simulink model "flash_model1"  (R2014b)
settings: Solver=FixedStepDiscrete  SolverMode=SingleTasking  StartTime=0.0  StopTime=10.0  FixedStep=.1  RelTol=1e-3
settings Model: SimulationMode=external  Creator=wildcat  LastModifiedBy=aodell
settings DataIOCC: SaveOutput=off  SignalLogging=off  SaveTime=off
settings SFSimCC: SimCustomHeaderCode=|
  | #include "/Users/aodell/Google Drive/Documents/MATLAB/test_sim/mycfiles/motorboard.h"
  | #include "/Users/aodell/Google Drive/Documents/MATLAB/test_sim/mycfiles/mot.h"
  | #include "/Users/aodell/Google Drive/Documents/MATLAB/test_sim/mycfiles/util.h"
  | #include "/Users/aodell/Google Drive/Documents/MATLAB/test_sim/mycfiles/gpio.h"
  | #include "/Users/aodell/Google Drive/Documents/MATLAB/test_sim/mycfiles/type.h"
settings SFSimCC: SimUserSources=|
  | "/Users/aodell/Google Drive/Documents/MATLAB/test_sim/mycfiles/motorboard.c"
  | "/Users/aodell/Google Drive/Documents/MATLAB/test_sim/mycfiles/mot.c"
  | "/Users/aodell/Google Drive/Documents/MATLAB/test_sim/mycfiles/util.c"
  | "/Users/aodell/Google Drive/Documents/MATLAB/test_sim/mycfiles/gpio.c"
settings RTWCC: GenCodeOnly=on  TargetLang=C++
settings GRTTargetCC: MatFileLogging=off  ExtMode=on  ExtModeMexArgs='192.168.1.1' 1 17725

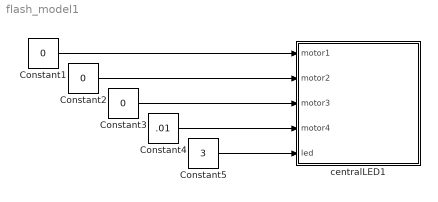
== system flash_model1 ==
  Constant1 : Constant  Value=0
  Constant2 : Constant  Value=0
  Constant3 : Constant  Value=0
  Constant4 : Constant  Value=.01
  Constant5 : Constant  Value=3
  centralLED1 : MATLAB Function  TreatAsAtomicUnit=on
  wires:
  Constant1/1 -> centralLED1/1(motor1)
  Constant2/1 -> centralLED1/2(motor2)
  Constant3/1 -> centralLED1/3(motor3)
  Constant4/1 -> centralLED1/4(motor4)
  Constant5/1 -> centralLED1/5(led)

== matlab function flash_model1/centralLED1 ==
  data: motor1 input; motor2 input; motor3 input; motor4 input; led input
function motorController(motor1,motor2,motor3,motor4,led)
%#codegen

persistent flag

coder.cinclude('/Users/aodell/Documents/MATLAB/test_sim/mycfiles/mot.h');
coder.cinclude('/Users/aodell/Documents/MATLAB/test_sim/mycfiles/motorboard.h');
coder.cinclude('/Users/aodell/Documents/MATLAB/test_sim/mycfiles/util.h');
coder.cinclude('/Users/aodell/Documents/MATLAB/test_sim/mycfiles/gpio.h');

switch coder.target

    % Define how the block behaves in simulation mode 
    case 'sfun' 

    % Define how the block behaves in real time execution 
    case 'rtw'
        
        if isempty(flag),
            coder.ceval('mot_Init');
            flag=1;
        end;
        
        motorArr= double([motor1,motor2,motor3,motor4]);
        coder.ceval('mot_Run',motorArr(1),motorArr(2),motorArr(3),motorArr(4));
        coder.ceval('mot_SetLeds',led,led,led,led);
        
end
